simulink model "Test_model_Function"  (R2024a)
settings: Solver=VariableStepAuto  StartTime=0.0  StopTime=inf  RelTol=1e-3
undefined symbols (not defined in the file or in its folder): X, Y, Z
libraries: sm_lib x62, nesl_utility x21, robotcorelib x4
(part 3 of 3)

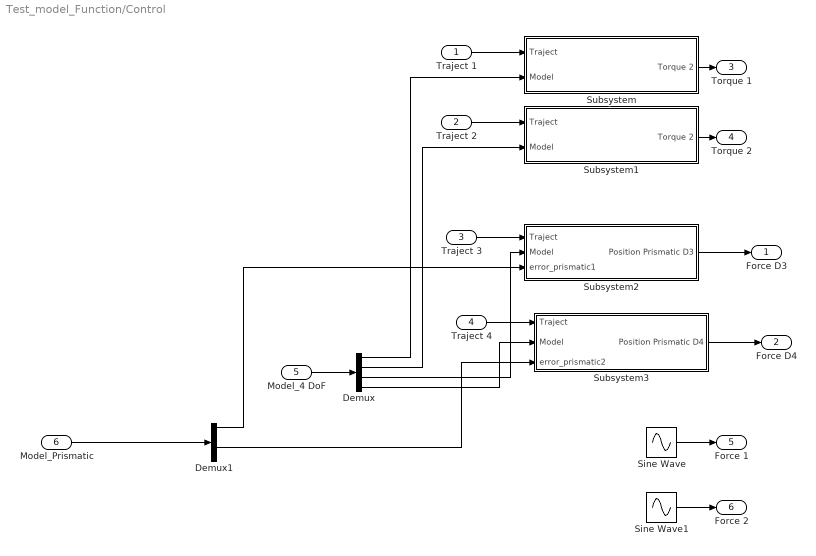
== system Test_model_Function/Control ==
  Traject 1 : Inport
  Traject 2 : Inport  Port=2
  Traject 3 : Inport  Port=3
  Traject 4 : Inport  Port=4
  Model_4 DoF : Inport  Port=5
  Model_Prismatic : Inport  Port=6
  Demux : Demux
  Demux1 : Demux
  Sine Wave : Sin  SampleTime=0
  Sine Wave1 : Sin  SampleTime=0
  Subsystem : Subsystem
  Subsystem1 : Subsystem
  Subsystem2 : Subsystem
  Subsystem3 : Subsystem
  Force D3 : Outport
  Force D4 : Outport  Port=2
  Torque 1 : Outport  Port=3
  Torque 2 : Outport  Port=4
  Force 1 : Outport  Port=5
  Force 2 : Outport  Port=6
  wires:
  Subsystem1/1(Torque 2) -> Torque 2/1
  Subsystem/1(Torque 2) -> Torque 1/1
  Subsystem3/1(Position Prismatic D4) -> Force D4/1
  Subsystem2/1(Position Prismatic D3) -> Force D3/1
  Model_4 DoF/1 -> Demux/1
  Demux/1 -> Subsystem/2(Model)
  Demux/2 -> Subsystem1/2(Model)
  Demux/3 -> Subsystem2/2(Model)
  Demux/4 -> Subsystem3/2(Model)
  Sine Wave/1 -> Force 1/1
  Sine Wave1/1 -> Force 2/1
  Traject 1/1 -> Subsystem/1(Traject)
  Traject 2/1 -> Subsystem1/1(Traject)
  Traject 3/1 -> Subsystem2/1(Traject)
  Traject 4/1 -> Subsystem3/1(Traject)
  Model_Prismatic/1 -> Demux1/1
  Demux1/1 -> Subsystem2/3(error_prismatic1)
  Demux1/3 -> Subsystem3/3(error_prismatic2)

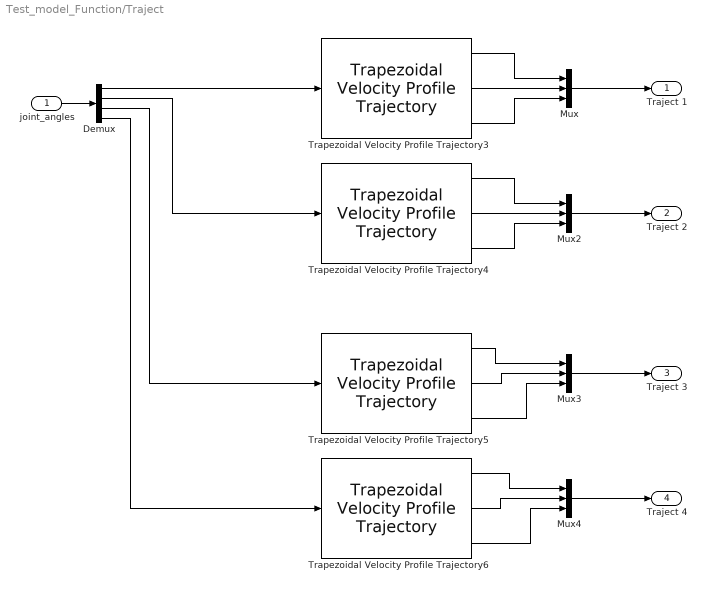
== system Test_model_Function/Traject ==
  joint_angles : Inport
  Demux : Demux
  Mux{,2..4} (4 alike) : Mux  Inputs=3
  Trapezoidal Velocity Profile Trajectory3 : robotcorelib/Trapezoidal Velocity Profile Trajectory  WaypointSource=Internal  Waypoints=[ 0, 0, 0]  NumParams=0  Parameter1=Peak Velocity  Parameter2=End Time  ParameterSource=Internal  PeakVelocity=[ 2; 2 ]  Acceleration=[ 1; 2 ]  EndTime=[ 1; 1 ]  AccelTime=[ 1; 2 ]  SimulateUsing=Interpreted execution
  Trapezoidal Velocity Profile Trajectory4 : robotcorelib/Trapezoidal Velocity Profile Trajectory  WaypointSource=Internal  Waypoints=[ 0, 0, 0]  NumParams=0  Parameter1=Peak Velocity  Parameter2=End Time  ParameterSource=Internal  PeakVelocity=[ 2; 2 ]  Acceleration=[ 1; 2 ]  EndTime=[ 1; 1 ]  AccelTime=[ 1; 2 ]  SimulateUsing=Interpreted execution
  Trapezoidal Velocity Profile Trajectory5 : robotcorelib/Trapezoidal Velocity Profile Trajectory  WaypointSource=Internal  Waypoints=[ 0, 1, 5]  NumParams=0  Parameter1=Peak Velocity  Parameter2=End Time  ParameterSource=Internal  PeakVelocity=[ 2; 2 ]  Acceleration=[ 1; 2 ]  EndTime=[ 1; 1 ]  AccelTime=[ 1; 2 ]  SimulateUsing=Interpreted execution
  Trapezoidal Velocity Profile Trajectory6 : robotcorelib/Trapezoidal Velocity Profile Trajectory  WaypointSource=Internal  Waypoints=[ 0, 1, 3]  NumParams=0  Parameter1=Peak Velocity  Parameter2=End Time  ParameterSource=Internal  PeakVelocity=[ 2; 2 ]  Acceleration=[ 1; 2 ]  EndTime=[ 1; 1 ]  AccelTime=[ 1; 2 ]  SimulateUsing=Interpreted execution
  Traject 1 : Outport
  Traject 2 : Outport  Port=2
  Traject 3 : Outport  Port=3
  Traject 4 : Outport  Port=4
  wires:
  Trapezoidal Velocity Profile Trajectory5/2 -> Mux3/2
  Trapezoidal Velocity Profile Trajectory3/2 -> Mux/2
  Trapezoidal Velocity Profile Trajectory6/1 -> Mux4/1
  Trapezoidal Velocity Profile Trajectory6/2 -> Mux4/2
  Trapezoidal Velocity Profile Trajectory3/3 -> Mux/3
  Trapezoidal Velocity Profile Trajectory6/3 -> Mux4/3
  Trapezoidal Velocity Profile Trajectory5/3 -> Mux3/3
  Trapezoidal Velocity Profile Trajectory3/1 -> Mux/1
  Trapezoidal Velocity Profile Trajectory4/3 -> Mux2/3
  Trapezoidal Velocity Profile Trajectory4/1 -> Mux2/1
  Trapezoidal Velocity Profile Trajectory4/2 -> Mux2/2
  Trapezoidal Velocity Profile Trajectory5/1 -> Mux3/1
  Mux/1 -> Traject 1/1
  joint_angles/1 -> Demux/1
  Demux/1 -> Trapezoidal Velocity Profile Trajectory3/1
  Demux/2 -> Trapezoidal Velocity Profile Trajectory4/1
  Demux/3 -> Trapezoidal Velocity Profile Trajectory5/1
  Demux/4 -> Trapezoidal Velocity Profile Trajectory6/1
  Mux2/1 -> Traject 2/1
  Mux3/1 -> Traject 3/1
  Mux4/1 -> Traject 4/1

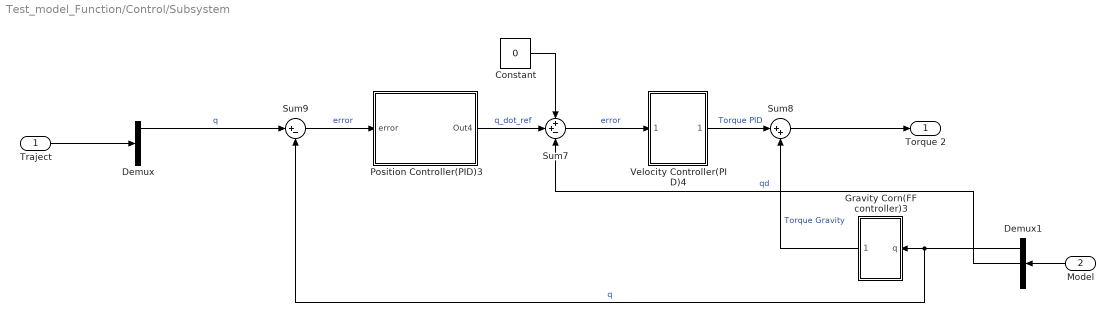
== system Test_model_Function/Control/Subsystem ==
  Traject : Inport
  Model : Inport  Port=2
  Constant : Constant  Value=0
  Demux : Demux  Outputs=3
  Demux1 : Demux  Outputs=3
  Gravity Corn(FF controller)3 : Subsystem
  Position Controller(PID)3 : Subsystem
  Sum7 : Sum  Inputs=++-
  Sum8 : Sum  Inputs=|++
  Sum9 : Sum  Inputs=|+-
  Velocity Controller(PID)4 : Subsystem
  Torque 2 : Outport
  wires:
  Position Controller(PID)3/1(Out4) -> Sum7/2  "q_dot_ref"
  Gravity Corn(FF controller)3/1(Out1) -> Sum8/2  "Torque Gravity"
  Traject/1 -> Demux/1
  Velocity Controller(PID)4/1(Out4) -> Sum8/1  "Torque PID"
  Sum7/1 -> Velocity Controller(PID)4/1(error)  "error"
  Sum9/1 -> Position Controller(PID)3/1(error)  "error"
  Sum8/1 -> Torque 2/1
  Model/1 -> Demux1/1
  Demux1/1 -> Sum9/2, Gravity Corn(FF controller)3/1(q)  "q"
  Demux1/2 -> Sum7/3  "qd"
  Constant/1 -> Sum7/1
  Demux/1 -> Sum9/1  "q"

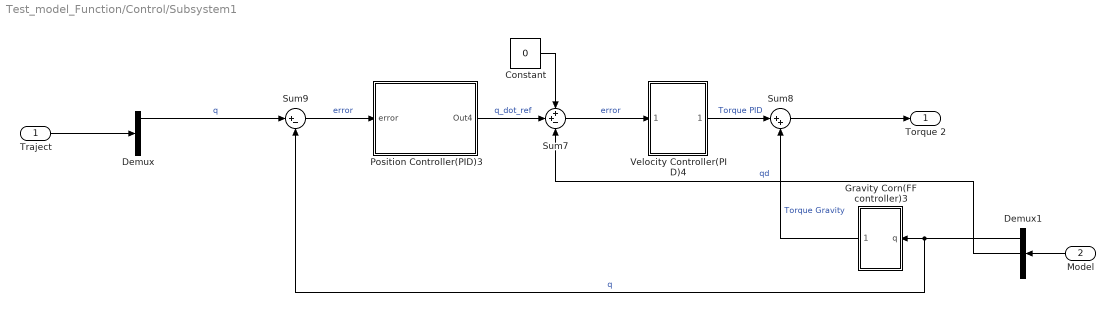
== system Test_model_Function/Control/Subsystem1 ==
  Traject : Inport
  Model : Inport  Port=2
  Constant : Constant  Value=0
  Demux : Demux  Outputs=3
  Demux1 : Demux  Outputs=3
  Gravity Corn(FF controller)3 : Subsystem
  Position Controller(PID)3 : Subsystem
  Sum7 : Sum  Inputs=++-
  Sum8 : Sum  Inputs=|++
  Sum9 : Sum  Inputs=|+-
  Velocity Controller(PID)4 : Subsystem
  Torque 2 : Outport
  wires:
  Position Controller(PID)3/1(Out4) -> Sum7/2  "q_dot_ref"
  Gravity Corn(FF controller)3/1(Out1) -> Sum8/2  "Torque Gravity"
  Traject/1 -> Demux/1
  Velocity Controller(PID)4/1(Out4) -> Sum8/1  "Torque PID"
  Sum7/1 -> Velocity Controller(PID)4/1(error)  "error"
  Sum9/1 -> Position Controller(PID)3/1(error)  "error"
  Sum8/1 -> Torque 2/1
  Model/1 -> Demux1/1
  Demux1/1 -> Sum9/2, Gravity Corn(FF controller)3/1(q)  "q"
  Demux1/2 -> Sum7/3  "qd"
  Constant/1 -> Sum7/1
  Demux/1 -> Sum9/1  "q"

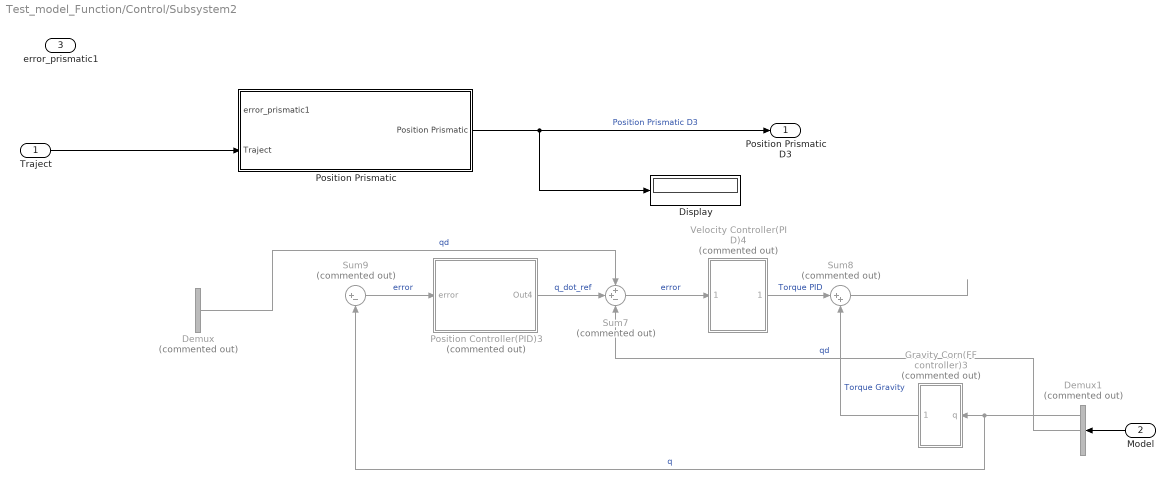
== system Test_model_Function/Control/Subsystem2 ==
  Traject : Inport
  Model : Inport  Port=2
  error_prismatic1 : Inport  Port=3
  Demux : Demux  Commented=on  Outputs=3
  Demux1 : Demux  Commented=on  Outputs=3
  Display : Display
  Gravity Corn(FF controller)3 : Subsystem  Commented=on
  Position Controller(PID)3 : Subsystem  Commented=on
  "Position Prismatic " : Subsystem
  Sum7 : Sum  Commented=on  Inputs=++-
  Sum8 : Sum  Commented=on  Inputs=|++
  Sum9 : Sum  Commented=on  Inputs=|+-
  Velocity Controller(PID)4 : Subsystem  Commented=on
  Position Prismatic D3 : Outport
  wires:
  Position Controller(PID)3/1(Out4) -> Sum7/2  "q_dot_ref"
  Gravity Corn(FF controller)3/1(Out1) -> Sum8/2  "Torque Gravity"
  Traject/1 -> "Position Prismatic "/2(Traject)
  Velocity Controller(PID)4/1(Out4) -> Sum8/1  "Torque PID"
  Sum7/1 -> Velocity Controller(PID)4/1(error)  "error"
  Sum9/1 -> Position Controller(PID)3/1(error)  "error"
  Sum8/1 -> ?
  Demux/2 -> Sum7/1  "qd"
  Model/1 -> Demux1/1
  Demux1/1 -> Sum9/2, Gravity Corn(FF controller)3/1(q)  "q"
  Demux1/2 -> Sum7/3  "qd"
  "Position Prismatic "/1(Position Prismatic) -> Display/1, Position Prismatic D3/1  "Position Prismatic D3"

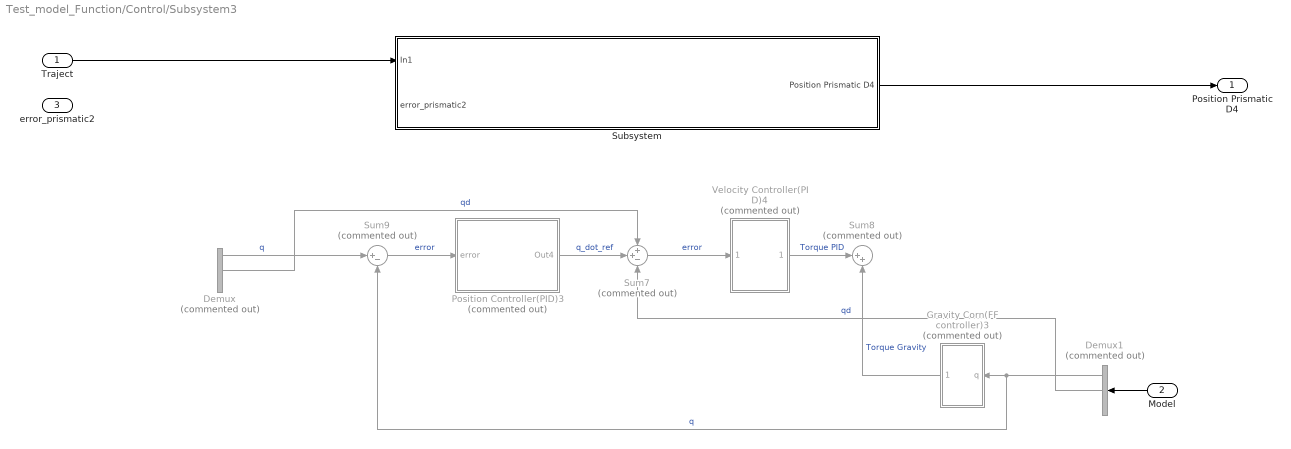
== system Test_model_Function/Control/Subsystem3 ==
  Traject : Inport
  Model : Inport  Port=2
  error_prismatic2 : Inport  Port=3
  Demux : Demux  Commented=on  Outputs=3
  Demux1 : Demux  Commented=on  Outputs=3
  Gravity Corn(FF controller)3 : Subsystem  Commented=on
  Position Controller(PID)3 : Subsystem  Commented=on
  Subsystem : Subsystem
  Sum7 : Sum  Commented=on  Inputs=++-
  Sum8 : Sum  Commented=on  Inputs=|++
  Sum9 : Sum  Commented=on  Inputs=|+-
  Velocity Controller(PID)4 : Subsystem  Commented=on
  Position Prismatic D4 : Outport
  wires:
  Position Controller(PID)3/1(Out4) -> Sum7/2  "q_dot_ref"
  Gravity Corn(FF controller)3/1(Out1) -> Sum8/2  "Torque Gravity"
  Velocity Controller(PID)4/1(Out4) -> Sum8/1  "Torque PID"
  Sum7/1 -> Velocity Controller(PID)4/1(error)  "error"
  Sum9/1 -> Position Controller(PID)3/1(error)  "error"
  Demux/1 -> Sum9/1  "q"
  Demux/2 -> Sum7/1  "qd"
  Model/1 -> Demux1/1
  Demux1/1 -> Sum9/2, Gravity Corn(FF controller)3/1(q)  "q"
  Demux1/2 -> Sum7/3  "qd"
  Traject/1 -> Subsystem/1(In1)
  Subsystem/1(Position Prismatic D4) -> Position Prismatic D4/1

== system Test_model_Function/Control/Subsystem/Gravity Corn(FF controller)3 ==
  note: mgLsin(zeta)
  q : Inport
  Sin : Trigonometry
  mg : Gain  Gain=1*9.80665*1
  Out1 : Outport
  wires:
  Sin/1 -> mg/1
  q/1 -> Sin/1
  mg/1 -> Out1/1

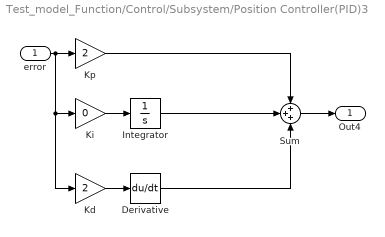
== system Test_model_Function/Control/Subsystem/Position Controller(PID)3 ==
  error : Inport
  Derivative : Derivative
  Integrator : Integrator
  Kd : Gain  Gain=2
  Ki : Gain  Gain=0
  Kp : Gain  Gain=2
  Sum : Sum  Inputs=+++
  Out4 : Outport
  wires:
  Derivative/1 -> Sum/3
  Ki/1 -> Integrator/1
  Integrator/1 -> Sum/2
  Kd/1 -> Derivative/1
  Kp/1 -> Sum/1
  error/1 -> Kd/1, Ki/1, Kp/1
  Sum/1 -> Out4/1

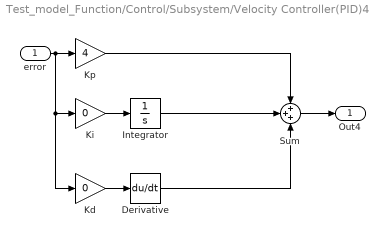
== system Test_model_Function/Control/Subsystem/Velocity Controller(PID)4 ==
  error : Inport
  Derivative : Derivative
  Integrator : Integrator
  Kd : Gain  Gain=0
  Ki : Gain  Gain=0
  Kp : Gain  Gain=4
  Sum : Sum  Inputs=+++
  Out4 : Outport
  wires:
  Derivative/1 -> Sum/3
  Ki/1 -> Integrator/1
  Integrator/1 -> Sum/2
  Kd/1 -> Derivative/1
  Kp/1 -> Sum/1
  error/1 -> Kd/1, Ki/1, Kp/1
  Sum/1 -> Out4/1

== system Test_model_Function/Control/Subsystem1/Gravity Corn(FF controller)3 ==
  note: mgLsin(zeta)
  q : Inport
  Sin : Trigonometry
  mg : Gain  Gain=1*9.80665*1
  Out1 : Outport
  wires:
  Sin/1 -> mg/1
  q/1 -> Sin/1
  mg/1 -> Out1/1

== system Test_model_Function/Control/Subsystem1/Position Controller(PID)3 ==
  error : Inport
  Derivative : Derivative
  Integrator : Integrator
  Kd : Gain  Gain=2
  Ki : Gain  Gain=0
  Kp : Gain  Gain=2
  Sum : Sum  Inputs=+++
  Out4 : Outport
  wires:
  Derivative/1 -> Sum/3
  Ki/1 -> Integrator/1
  Integrator/1 -> Sum/2
  Kd/1 -> Derivative/1
  Kp/1 -> Sum/1
  error/1 -> Kd/1, Ki/1, Kp/1
  Sum/1 -> Out4/1

== system Test_model_Function/Control/Subsystem1/Velocity Controller(PID)4 ==
  error : Inport
  Derivative : Derivative
  Integrator : Integrator
  Kd : Gain  Gain=0
  Ki : Gain  Gain=0
  Kp : Gain  Gain=4
  Sum : Sum  Inputs=+++
  Out4 : Outport
  wires:
  Derivative/1 -> Sum/3
  Ki/1 -> Integrator/1
  Integrator/1 -> Sum/2
  Kd/1 -> Derivative/1
  Kp/1 -> Sum/1
  error/1 -> Kd/1, Ki/1, Kp/1
  Sum/1 -> Out4/1

== system Test_model_Function/Control/Subsystem2/Gravity Corn(FF controller)3 ==
  note: mgLsin(zeta)
  q : Inport
  Sin : Trigonometry
  mg : Gain  Gain=1*9.80665*1
  Out1 : Outport
  wires:
  Sin/1 -> mg/1
  q/1 -> Sin/1
  mg/1 -> Out1/1

== system Test_model_Function/Control/Subsystem2/Position Controller(PID)3 ==
  error : Inport
  Derivative : Derivative
  Integrator : Integrator
  Kd : Gain  Gain=2
  Ki : Gain  Gain=0
  Kp : Gain  Gain=2
  Sum : Sum  Inputs=+++
  Out4 : Outport
  wires:
  Derivative/1 -> Sum/3
  Ki/1 -> Integrator/1
  Integrator/1 -> Sum/2
  Kd/1 -> Derivative/1
  Kp/1 -> Sum/1
  error/1 -> Kd/1, Ki/1, Kp/1
  Sum/1 -> Out4/1

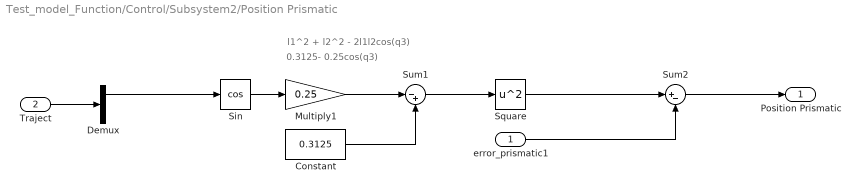
== system Test_model_Function/Control/Subsystem2/Position Prismatic  ==
  note: l1^2 + l2^2 - 2l1l2cos(q3)
  note: 0.3125- 0.25cos(q3)
  error_prismatic1 : Inport
  Traject : Inport  Port=2
  Constant : Constant  Value=0.3125
  Demux : Demux  Outputs=3
  Multiply1 : Gain  Gain=0.25
  Sin : Trigonometry  Operator=cos
  Square : Math  Operator=square
  Sum1 : Sum  Inputs=|-+
  Sum2 : Sum  Inputs=|+-
  Position Prismatic : Outport
  wires:
  Sum1/1 -> Square/1
  Square/1 -> Sum2/1
  Constant/1 -> Sum1/2
  Sin/1 -> Multiply1/1
  error_prismatic1/1 -> Sum2/2
  Sum2/1 -> Position Prismatic/1
  Traject/1 -> Demux/1
  Multiply1/1 -> Sum1/1
  Demux/1 -> Sin/1

== system Test_model_Function/Control/Subsystem2/Velocity Controller(PID)4 ==
  error : Inport
  Derivative : Derivative
  Integrator : Integrator
  Kd : Gain  Gain=0
  Ki : Gain  Gain=0
  Kp : Gain  Gain=4
  Sum : Sum  Inputs=+++
  Out4 : Outport
  wires:
  Derivative/1 -> Sum/3
  Ki/1 -> Integrator/1
  Integrator/1 -> Sum/2
  Kd/1 -> Derivative/1
  Kp/1 -> Sum/1
  error/1 -> Kd/1, Ki/1, Kp/1
  Sum/1 -> Out4/1

== system Test_model_Function/Control/Subsystem3/Gravity Corn(FF controller)3 ==
  note: mgLsin(zeta)
  q : Inport
  Sin : Trigonometry
  mg : Gain  Gain=1*9.80665*1
  Out1 : Outport
  wires:
  Sin/1 -> mg/1
  q/1 -> Sin/1
  mg/1 -> Out1/1

== system Test_model_Function/Control/Subsystem3/Position Controller(PID)3 ==
  error : Inport
  Derivative : Derivative
  Integrator : Integrator
  Kd : Gain  Gain=2
  Ki : Gain  Gain=0
  Kp : Gain  Gain=2
  Sum : Sum  Inputs=+++
  Out4 : Outport
  wires:
  Derivative/1 -> Sum/3
  Ki/1 -> Integrator/1
  Integrator/1 -> Sum/2
  Kd/1 -> Derivative/1
  Kp/1 -> Sum/1
  error/1 -> Kd/1, Ki/1, Kp/1
  Sum/1 -> Out4/1

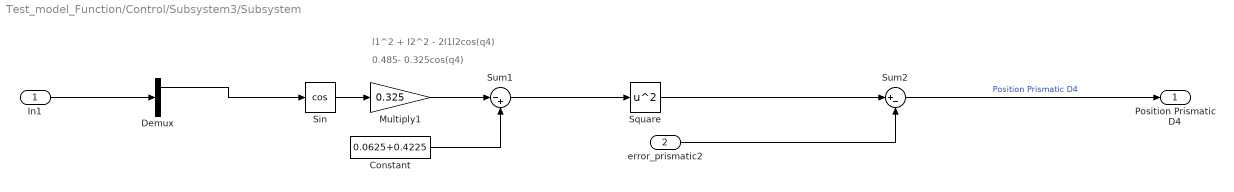
== system Test_model_Function/Control/Subsystem3/Subsystem ==
  note: l1^2 + l2^2 - 2l1l2cos(q4)
  note: 0.485- 0.325cos(q4)
  In1 : Inport
  error_prismatic2 : Inport  Port=2
  Constant : Constant  Value=0.0625+0.4225
  Demux : Demux  Outputs=3
  Multiply1 : Gain  Gain=0.325
  Sin : Trigonometry  Operator=cos
  Square : Math  Operator=square
  Sum1 : Sum  Inputs=|-+
  Sum2 : Sum  Inputs=|+-
  Position Prismatic D4 : Outport
  wires:
  Square/1 -> Sum2/1
  error_prismatic2/1 -> Sum2/2
  Sin/1 -> Multiply1/1
  Multiply1/1 -> Sum1/1
  Sum2/1 -> Position Prismatic D4/1  "Position Prismatic D4"
  Constant/1 -> Sum1/2
  Sum1/1 -> Square/1
  In1/1 -> Demux/1
  Demux/1 -> Sin/1

== system Test_model_Function/Control/Subsystem3/Velocity Controller(PID)4 ==
  error : Inport
  Derivative : Derivative
  Integrator : Integrator
  Kd : Gain  Gain=0
  Ki : Gain  Gain=0
  Kp : Gain  Gain=4
  Sum : Sum  Inputs=+++
  Out4 : Outport
  wires:
  Derivative/1 -> Sum/3
  Ki/1 -> Integrator/1
  Integrator/1 -> Sum/2
  Kd/1 -> Derivative/1
  Kp/1 -> Sum/1
  error/1 -> Kd/1, Ki/1, Kp/1
  Sum/1 -> Out4/1

== matlab function Test_model_Function/MATLAB Function1 ==
  data: joint_angles input; x output; y output; z output; phi output
function [x, y, z, phi] = FK_Simulink(joint_angles)
    % FK_Simulink: Calculates the position and orientation of the end effector for a 4-DOF manipulator

    % Lengths of the links
    L1 = 0.25; % Link 1
    L2 = 1; % Link 2
    L3 = 1.5; % Link 3
    L4 = 0.75; % Link 4 (End Effector)

    % Extract joint angles
    q1 = joint_angles(1); % Joint 1 (base rotation)
    q2 = joint_angles(2); % Joint 2 (shoulder rotation)
    q3 = joint_angles(3); % Joint 3 (elbow rotation)
    q4 = joint_angles(4); % Joint 4 (end effector orientation)

    % Transformation Matrices
    % Transform from base frame to end effector
    % Transformation for Joint 1 (Rotation around the base)
    T1 = [cos(q1), -sin(q1), 0, 0;
          sin(q1), cos(q1), 0, 0;
          0, 0, 1, L1;
          0, 0, 0, 1];

    % Transformation for Joint 2 (shoulder)
    T2 = [cos(q2), -sin(q2), 0, 0;
           0, 0, -1, 0;
          sin(q2), cos(q2), 0, 0;
          0, 0, 0, 1];

    % Transformation for Joint 3 (elbow)
    T3 = [cos(q3), -sin(q3), 0, L2;
          sin(q3), cos(q3), 0, 0;
          0, 0, 1, 0;
          0, 0, 0, 1];

    % Transformation for Joint 4 (end effector orientation)
    T4 = [cos(q4), -sin(q4), 0, L3;
          sin(q4), cos(q4), 0, 0;
          0, 0, 1, 0;
          0, 0, 0, 1];

    T5 = [1, 0, 0, L4;
      0, 1, 0, 0;
      0, 0, 1, 0;
      0, 0, 0, 1];

    % Final transformation from the base to end effector
    T = T1 * T2 * T3 * T4 * T5;

    % Extract position from the final transformation matrix
    x = T(1, 4); % x-position of the end effector
    y = T(2, 4); % y-position of the end effector
    z = T(3, 4); % z-position of the end effector

    % Extract orientation (phi) from the transformation matrix
    phi = atan2(T(2, 1), T(1, 1)); % Rotation around the z-axis (orientation of the end effector)
end

== matlab function Test_model_Function/MATLAB Function ==
  data: x input; joint_angles output; y input; z input; phi input
function joint_angles = IK_Simulink(x, y, z, phi)
    % IK_Simulink: Calculates joint angles and displacements for a 4-DOF manipulator (RRPP)
    
    % Lengths of the links
    L1 = 0.25; % Link 1 (base)
    L2 = 1; % Link 2
    L3 = 1.5; % Link 3
    L4 = 0.75; % Link 4 (End Effector)
    
    % 1. Calculate q1 (base rotation)
    q1 = atan2(y, x); % Base rotation angle
    
    % Project the target onto the xy-plane
    xe = sqrt(x^2 + y^2); % Projected target on the xy-plane
    ze = z - L1; % Remove L1 to focus on the target in the xy-plane

    % 2. Calculate the distance between joint 2 and the target (xe, ze)
    r = sqrt(xe^2 + ze^2);
    
    % Check if the target is within reach
    if r > (L2 + L3 + L4)
        error('Target position is out of reach.');
    end
    
    % 3. Use the Law of Cosines to calculate q2 (shoulder joint)
    cos_theta2 = (r^2 - L2^2 - L3^2) / (2 * L2 * L3);
    q3 = atan2(-sqrt(1 - cos_theta2^2), cos_theta2); % Elbow-down configuration
    
    % 4. Calculate q2 (shoulder joint)
    beta = atan2(ze, xe); % Angle between the target and joint 2
    alpha = atan2(L3 * sin(q3), L2 + L3 * cos(q3)); % Angle from L2 to L3
    q2 = beta - alpha; % Final angle for joint 2
    
    % 5. For Prismatic Joints:
    % Calculate q3 (Prismatic joint displacement) along the x-axis (P1)
    q3 = r - L2; % Displacement required to position the prismatic joint along x
    
    % 6. Calculate q4 (Prismatic joint displacement) along the z-axis (P2)
    q4 = ze - L3; % Displacement required to position the prismatic joint along z

    % 7. Calculate q5 (End effector orientation)
    q5 = phi - (q2 + q3); % End effector rotation
    
    % Return joint angles and displacements as a vector
    joint_angles = [q1; q2; q3; q4]; % Now q3 and q4 are displacements (prismatic joints)
end

== matlab function Test_model_Function/MATLAB Function2 ==
  data: x input; joint_angles output; y input; z input
function joint_angles = IK_RRRR(x, y, z)
    % IK_RRRR: Calculates joint angles for a 4-DOF manipulator (RRRR)
    
    % Lengths of the links
    L1 = 0.25; % Link 1 (base)
    L2 = 1; % Link 2
    L3 = 1.5; % Link 3
    L4 = 0.75; % Link 4 (End Effector)

    % 1. Calculate q1 (base rotation)
    q1 = atan2(y, x); % Base rotation angle

    % Project the target onto the xy-plane
    xe = sqrt(x^2 + y^2); % Projected target on the xy-plane
    ze = z - L1; % Remove L1 to focus on the target in the xy-plane

    % 2. Calculate the distance between joint 2 and the target (xe, ze)
    r = sqrt(xe^2 + ze^2);
    
    % Check if the target is within reach
    if r > (L2 + L3 + L4)
        error('Target position is out of reach.');
    end
    
    % 3. Use the Law of Cosines to calculate q3 (elbow joint)
    cos_theta3 = (r^2 - L2^2 - L3^2 - L4^2) / (2 * L2 * L3); % Law of Cosines for q3
    q3 = atan2(-sqrt(1 - cos_theta3^2), cos_theta3); % Elbow-down configuration
    
    % 4. Calculate q2 (shoulder joint)
    beta = atan2(ze, xe); % Angle between the target and joint 2
    alpha = atan2(L3 * sin(q3), L2 + L3 * cos(q3)); % Angle from L2 to L3
    q2 = beta - alpha;

    % 5. Calculate q4 (wrist joint)
    % Angle between link L3 and the end effector orientation
    q4 = atan2(z - L1 - L4 * sin(q3), sqrt(x^2 + y^2));

    % Return the joint angles as a vector
    joint_angles = [q1, q2, q3, q4];
end

== matlab function Test_model_Function/MATLAB Function3 ==
  data: joint_angles input; x output; y output; z output
function [x, y, z] = FK_Simulink(joint_angles)
    % FK_Simulink: Calculates the position and orientation of the end effector for a 4-DOF manipulator

    % Lengths of the links
    L1 = 0.25; % Link 1
    L2 = 1; % Link 2
    L3 = 1.5; % Link 3
    L4 = 0.75; % Link 4 (End Effector)

    % Extract joint angles
    q1 = joint_angles(1); % Joint 1 (base rotation)
    q2 = joint_angles(2); % Joint 2 (shoulder rotation)
    q3 = joint_angles(3); % Joint 3 (elbow rotation)
    q4 = joint_angles(4); % Joint 4 (end effector orientation)

    % Transformation Matrices
    % Transform from base frame to end effector
    % Transformation for Joint 1 (Rotation around the base)
    T1 = [cos(q1), -sin(q1), 0, 0;
          sin(q1), cos(q1), 0, 0;
          0, 0, 1, L1;
          0, 0, 0, 1];

    % Transformation for Joint 2 (shoulder)
    T2 = [cos(q2), -sin(q2), 0, 0;
           0, 0, -1, 0;
          sin(q2), cos(q2), 0, 0;
          0, 0, 0, 1];

    % Transformation for Joint 3 (elbow)
    T3 = [cos(q3), -sin(q3), 0, L2;
          sin(q3), cos(q3), 0, 0;
          0, 0, 1, 0;
          0, 0, 0, 1];

    % Transformation for Joint 4 (end effector orientation)
    T4 = [cos(q4), -sin(q4), 0, L3;
          sin(q4), cos(q4), 0, 0;
          0, 0, 1, 0;
          0, 0, 0, 1];

    T5 = [1, 0, 0, L4;
      0, 1, 0, 0;
      0, 0, 1, 0;
      0, 0, 0, 1];

    % Final transformation from the base to end effector
    T = T1 * T2 * T3 * T4 * T5;

    % Extract position from the final transformation matrix
    x = T(1, 4); % x-position of the end effector
    y = T(2, 4); % y-position of the end effector
    z = T(3, 4); % z-position of the end effector

  
end

== matlab function Test_model_Function/MATLAB Function4 ==
  data: joint_angles input; x output; y output; z output
function [x, y, z] = FK_RRRR(joint_angles)
    % FK_RRRR: Forward Kinematics for a 4-DOF manipulator (RRRR) using DH parameters
    % Input: joint_angles - a vector of joint angles [q1, q2, q3, q4]
    % Output: x, y, z - position of the end effector
    
    % DH parameters for each joint (d, a, alpha, theta)
    L1 = 0.25; % Link 1 (base)
    L2 = 1;    % Link 2
    L3 = 1.5;  % Link 3
    L4 = 0.75; % Link 4 (End Effector)
    
    % Joint angles (q1, q2, q3, q4)
    q1 = joint_angles(1);
    q2 = joint_angles(2);
    q3 = joint_angles(3);
    q4 = joint_angles(4);
    
    % DH Transformation Matrices for each joint
    % Joint 1 (base rotation)
    T1 = [cos(q1), -sin(q1), 0, 0;
          sin(q1), cos(q1), 0, 0;
          0, 0, 1, L1;
          0, 0, 0, 1];
      
    % Joint 2 (shoulder joint, alpha = pi/2)
    T2 = [cos(q2), -sin(q2), 0, 0;
          sin(q2), cos(q2), 0, 0;
          0, 0, 1, 0;
          0, 0, 0, 1];
      
    % Joint 3 (elbow joint)
    T3 = [cos(q3), -sin(q3), 0, L2;
          sin(q3), cos(q3), 0, 0;
          0, 0, 1, 0;
          0, 0, 0, 1];
      
    % Joint 4 (wrist joint)
    T4 = [cos(q4), -sin(q4), 0, L3;
          sin(q4), cos(q4), 0, 0;
          0, 0, 1, 0;
          0, 0, 0, 1];
      
    % End Effector (End link)
    T5 = [1, 0, 0, L4;
          0, 1, 0, 0;
          0, 0, 1, 0;
          0, 0, 0, 1];
      
    % Compute the total transformation matrix by multiplying the individual transformations
    T = T1 * T2 * T3 * T4 * T5;
    
    % Extract the end effector position from the transformation matrix
    x = T(1, 4); % x position
    y = T(2, 4); % y position
    z = T(3, 4); % z position
end
